simulink model "open_loop_linear"  (R2018b)
settings: Solver=VariableStepAuto  StartTime=0.0  StopTime=10.0  RelTol=1e-3
undefined symbols (not defined in the file or in its folder): system
settings Model: Creator=BARIS  LastModifiedBy=BARIS

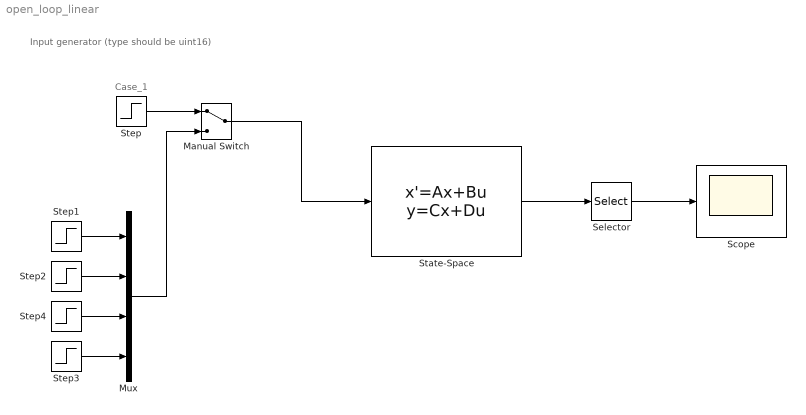
== system open_loop_linear ==
  note: Case_1
  note: Input generator
      | (type should be uint16)
  Manual Switch : ManualSwitch
  Mux : Mux
  Scope : Scope
  Selector : Selector  InputPortWidth=15  IndexOptions=Index vector (dialog)  Indices=[5:12]  OutputSizes=1
  State-Space : StateSpace  A=system.A  B=system.B  C=system.C  D=system.D  InitialCondition=0
  Step : Step  Time=4  Before=[0;0;0;0]  After=[10;10;0;0]  SampleTime=0
  Step1 : Step  Time=4  After=1000  SampleTime=0
  Step2 : Step  Time=0  After=0  SampleTime=0
  Step3 : Step  Time=0  After=0  SampleTime=0
  Step4 : Step  Time=6  After=2000  SampleTime=0
  wires:
  Step3/1 -> Mux/4
  Step4/1 -> Mux/3
  Step/1 -> Manual Switch/1
  Step1/1 -> Mux/1
  Mux/1 -> Manual Switch/2
  Step2/1 -> Mux/2
  Manual Switch/1 -> State-Space/1
  State-Space/1 -> Selector/1
  Selector/1 -> Scope/1
